simulink model "scalemodelsimulation"  (R2019b)
settings: Solver=ode15s  StartTime=0.0  StopTime=100  FixedStep=0.05  MaxStep=0.5  MinStep=0.01  RelTol=1e-1  AbsTol=1e-1
values from neighbouring files (symbols this model uses):
  x0 = [0, 0, 0.05, 2, 0, 0.01, 0.02, 0, 0, 0, 0, 0]    [createmodels.m]    (also in pidcontrolstartupscript.m = [0, 0, 0.05, 8, 0, 0.01, 0.02, 0, 0, 0, 0, 0])
undefined symbols (not defined in the file or in its folder): scalemodelstatefunction
libraries: mpclib x1, aerolibanim x1
settings Model: SimulationMode=accelerator  PacingRate=1000  Creator=Vlad  LastModifiedBy=Vlad
settings SolverCC: MaxConsecutiveMinStep=10
settings DataIOCC: ReturnWorkspaceOutputsName=tpe2155fcc_9c3f_42dd_9b90_435354f31060

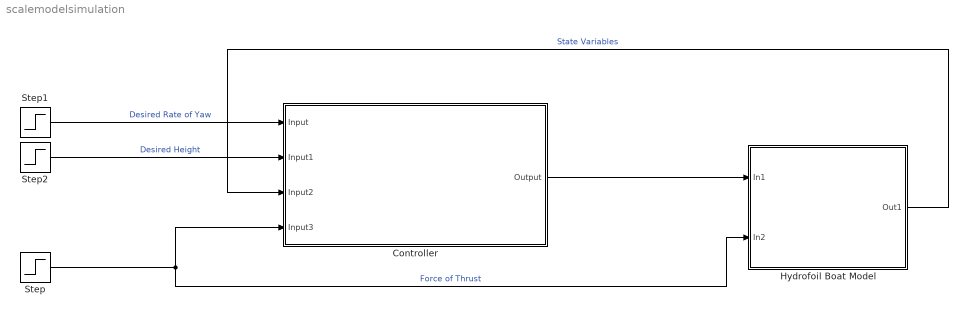
== system scalemodelsimulation ==
  Controller : Subsystem
  Hydrofoil Boat Model : Subsystem
  Step : Step  Time=0  After=35  SampleTime=0
  Step1 : Step  Time=0  After=0  SampleTime=0
  Step2 : Step  Time=0  After=2  SampleTime=0
  wires:
  Controller/1(Output) -> Hydrofoil Boat Model/1(In1)
  Hydrofoil Boat Model/1(Out1) -> Controller/3(Input2)  "State Variables"
  Step/1 -> Controller/4(Input3), Hydrofoil Boat Model/2(In2)  "Force of Thrust"
  Step1/1 -> Controller/1(Input)  "Desired Rate of Yaw"
  Step2/1 -> Controller/2(Input1)  "Desired Height"

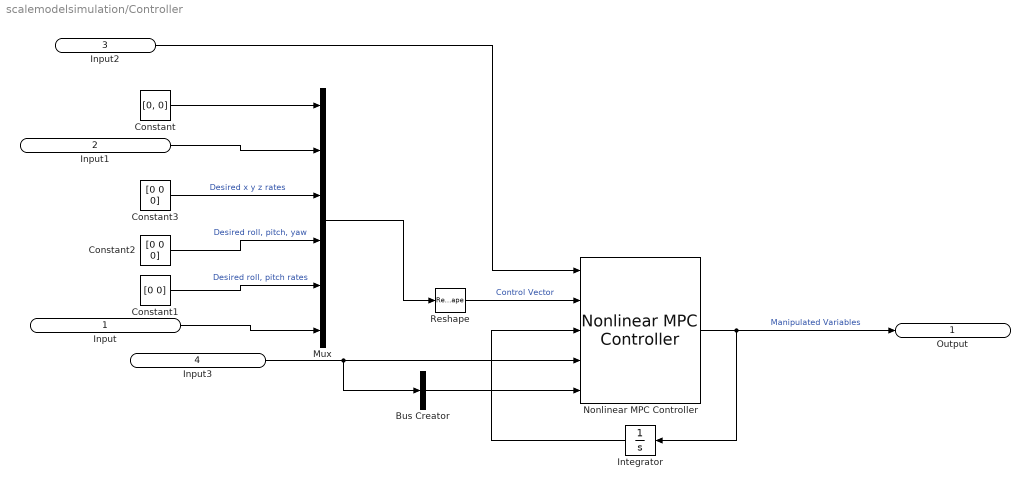
== system scalemodelsimulation/Controller ==
  Input : Inport
  Input1 : Inport  Port=2
  Input2 : Inport  Port=3
  Input3 : Inport  Port=4
  Bus Creator : BusCreator  Inputs=1  OutDataTypeStr=Bus: myBusObject_41  NonVirtualBus=on
      settings: InheritFromInputs=off
  Constant : Constant  Value=[0, 0]
  Constant1 : Constant  Value=[0 0]
  Constant2 : Constant  Value=[0 0 0]
  Constant3 : Constant  Value=[0 0 0]
  Integrator : Integrator
  Mux : Mux  Inputs=6
  Nonlinear MPC Controller : mpclib/Nonlinear MPC Controller  SCDEnableBlockLinearizationSpecification=on  nlmpcobj=nlobj  UseObjectTs=on  md_enabled=on  mvtarget_enabled=off  param_enabled=on  cost_enabled=off  mvseq_enabled=off  stateseq_enabled=off  ovseq_enabled=off  slack_enabled=off  status_enabled=off  ov_min=off  ov_max=off  mv_min=off  mv_max=off  mvrate_min=off  mvrate_max=off  state_min=off  state_max=off  ov_weight=off  mv_weight=off  mvrate_weight=off  ecr_weight=off  nlp_initialize=off
      settings: SourceProductName=Model Predictive Control Toolbox
  Reshape : Reshape  OutputDimensionality=Row vector (2-D)
  Output : Outport
  wires:
  Nonlinear MPC Controller/1 -> Output/1, Integrator/1  "Manipulated Variables"
  Integrator/1 -> Nonlinear MPC Controller/3
  Reshape/1 -> Nonlinear MPC Controller/2  "Control Vector"
  Input2/1 -> Nonlinear MPC Controller/1
  Mux/1 -> Reshape/1
  Input3/1 -> Nonlinear MPC Controller/4, Bus Creator/1
  Bus Creator/1 -> Nonlinear MPC Controller/5
  Input1/1 -> Mux/2
  Constant/1 -> Mux/1
  Constant3/1 -> Mux/3  "Desired x y z rates"
  Input/1 -> Mux/6
  Constant2/1 -> Mux/4  "Desired roll, pitch, yaw"
  Constant1/1 -> Mux/5  "Desired roll, pitch rates"

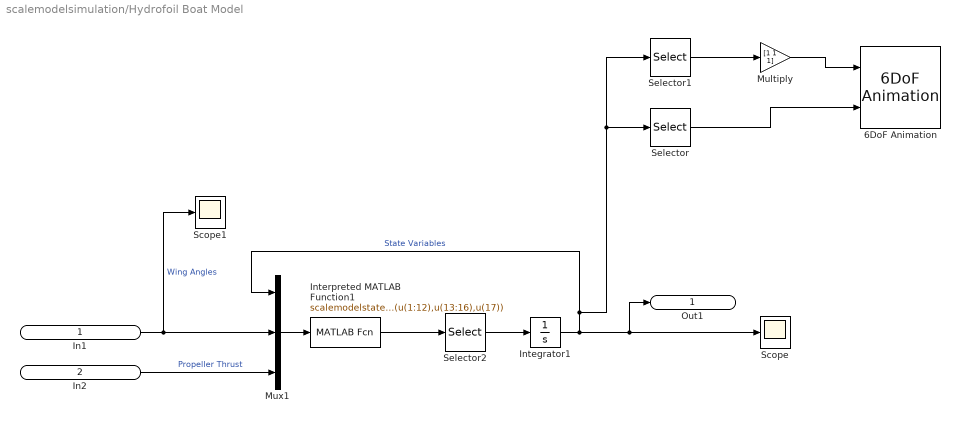
== system scalemodelsimulation/Hydrofoil Boat Model ==
  In1 : Inport
  In2 : Inport  Port=2
  6DoF Animation : aerolibanim/6DoF Animation  u1=[0 30 -2 2 -1 0]  u2=0.1  u3=5  u4=[4000 0 -5000]  u5=Fixed position  u6=[20 20 -20]  u7=20  u8=on
      settings: SourceProductName=Aerospace Blockset
  Integrator1 : Integrator  InitialCondition=x0
  Interpreted MATLAB Function1 : MATLABFcn  MATLABFcn=scalemodelstatefunction(u(1:12),u(13:16),u(17))  OutputDimensions=12
  Multiply : Gain  Gain=[1 1 1]
  Mux1 : Mux  Inputs=3
  Scope : Scope
  Scope1 : Scope
  Selector : Selector  InputPortWidth=12  IndexOptions=Index vector (dialog)  Indices=[8 7 9]  OutputSizes=1
  Selector1 : Selector  InputPortWidth=12  IndexOptions=Index vector (dialog)  Indices=[1 2 3]  OutputSizes=1
  Selector2 : Selector  InputPortWidth=12  IndexOptions=Index vector (dialog)  Indices=[1 2 3 4 5 6 7 8 9 10 11 12]  OutputSizes=1
  Out1 : Outport
  wires:
  Integrator1/1 -> Out1/1, Scope/1, Selector/1, Selector1/1, Mux1/1  "State Variables"
  Multiply/1 -> 6DoF Animation/1
  Selector1/1 -> Multiply/1
  Mux1/1 -> Interpreted MATLAB Function1/1
  Interpreted MATLAB Function1/1 -> Selector2/1
  Selector2/1 -> Integrator1/1
  Selector/1 -> 6DoF Animation/2
  In2/1 -> Mux1/3  "Propeller Thrust"
  In1/1 -> Scope1/1, Mux1/2  "Wing Angles"
